simulink model "lqg_regulator"  (R2016a)
settings: Solver=VariableStepAuto  StartTime=0.0  StopTime=10.0  RelTol=1e-3
values from neighbouring files (symbols this model uses):
  A = [   0 1 0 0 ... (first row only)    [calculation.m]
  B = [0;b2;0;b4]    [calculation.m]
  C = [0 1 0 0]    [calculation.m]
  G = -inv(Re)*B'*P12    [calculation.m]
undefined symbols (not defined in the file or in its folder): F, KI
settings Model: Creator=shohei  LastModifiedBy=shohei

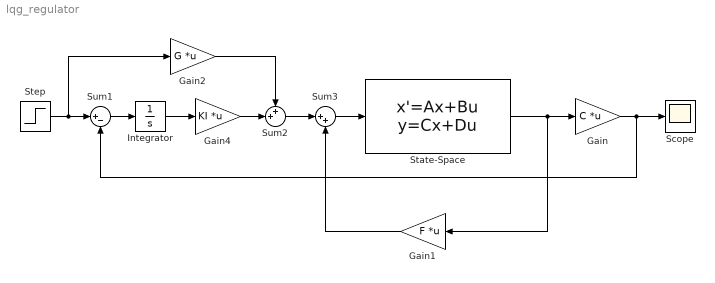
== system lqg_regulator ==
  Gain : Gain  Gain=C  Multiplication=Matrix(K*u)
  Gain1 : Gain  Gain=F  Multiplication=Matrix(K*u)
  Gain2 : Gain  Gain=G  Multiplication=Matrix(K*u)
  Gain4 : Gain  Gain=KI  Multiplication=Matrix(K*u)
  Integrator : Integrator
  Scope : Scope
  State-Space : StateSpace  A=A  B=B  C=eye(4)  D=[0; 0; 0; 0]  X0=0
  Step : Step  SampleTime=0
  Sum1 : Sum  Inputs=|+-
  Sum2 : Sum  Inputs=++|
  Sum3 : Sum  Inputs=|++
  wires:
  State-Space/1 -> Gain/1, Gain1/1
  Gain/1 -> Scope/1, Sum1/2
  Step/1 -> Gain2/1, Sum1/1
  Sum1/1 -> Integrator/1
  Integrator/1 -> Gain4/1
  Gain2/1 -> Sum2/1
  Gain4/1 -> Sum2/2
  Sum2/1 -> Sum3/1
  Gain1/1 -> Sum3/2
  Sum3/1 -> State-Space/1
